simulink library "Environment_ul"  (R2020a)
settings: Solver=VariableStepAuto  StartTime=0.0  StopTime=10.0  RelTol=1e-3
undefined symbols (not defined in the file): t_start, UNCC, x_f
libraries: simulink x1
settings Model: Creator=John Jr  LastModifiedBy=John Jr

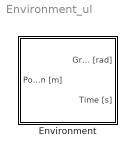
== system Environment_ul ==
  Environment : Subsystem

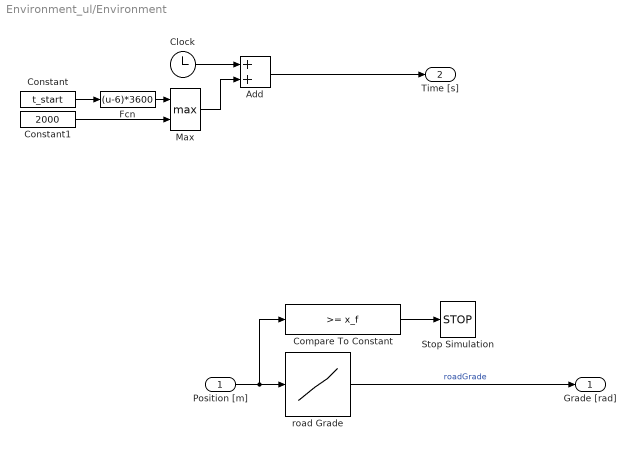
== system Environment_ul/Environment ==
  Position [m] : Inport
  Add : Sum
  Clock : Clock
      settings: Decimation=1/timeStep
  Compare To Constant : simulink/Logic and Bit Operations/Compare To Constant  relop=>=  const=x_f  OutDataTypeStr=boolean
  Constant : Constant  Value=t_start
  Constant1 : Constant  Value=2000
  Fcn : Fcn  Expr=(u-6)*3600
  Max : MinMax  Function=max  Inputs=2
  Stop Simulation : Stop
  road Grade : Lookup_n-D  NumberOfTableDimensions=1  BreakpointsForDimension1=UNCC.X_vec  Table=UNCC.theta_vec  InternalRulePriority=Speed  RndMeth=Simplest  InputSameDT=on
  Grade [rad] : Outport  VectorParamsAs1DForOutWhenUnconnected=off
  Time [s] : Outport  Port=2  VectorParamsAs1DForOutWhenUnconnected=off
  wires:
  Position [m]/1 -> Compare To Constant/1, road Grade/1
  road Grade/1 -> Grade [rad]/1  "roadGrade"
  Clock/1 -> Add/1
  Add/1 -> Time [s]/1
  Constant/1 -> Fcn/1
  Max/1 -> Add/2
  Fcn/1 -> Max/1
  Constant1/1 -> Max/2
  Compare To Constant/1 -> Stop Simulation/1
